simulink model "second_proto"  (R2023a)
settings: Solver=VariableStepAuto  StartTime=0.0  StopTime=10.0  RelTol=1e-3
settings Model: Creator=Алексей  LastModifiedBy=Алексей

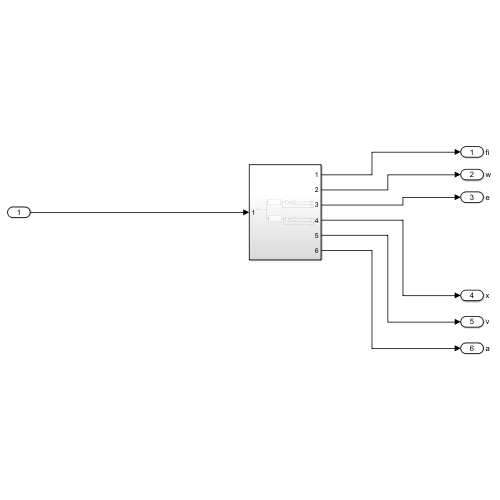
[thumbnail: Simulink's stored preview of the top-level diagram]
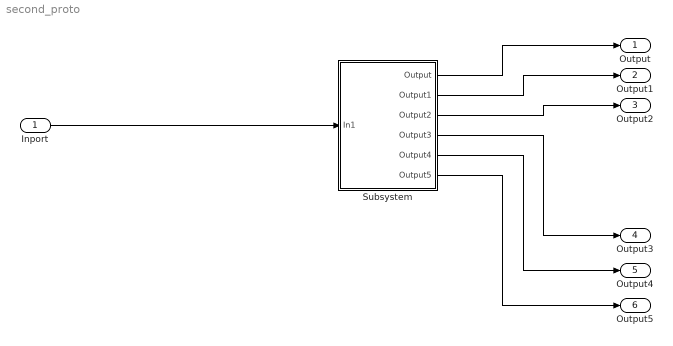
== system second_proto ==
  Inport : Inport
  Subsystem : Subsystem
  Output : Outport  SignalName=fi
  Output1 : Outport  Port=2  SignalName=w
  Output2 : Outport  Port=3  SignalName=e
  Output3 : Outport  Port=4  SignalName=x
  Output4 : Outport  Port=5  SignalName=v
  Output5 : Outport  Port=6  SignalName=a
  wires:
  Inport/1 -> Subsystem/1(In1)
  Subsystem/1(Output) -> Output/1
  Subsystem/2(Output1) -> Output1/1
  Subsystem/3(Output2) -> Output2/1
  Subsystem/4(Output3) -> Output3/1
  Subsystem/5(Output4) -> Output4/1
  Subsystem/6(Output5) -> Output5/1

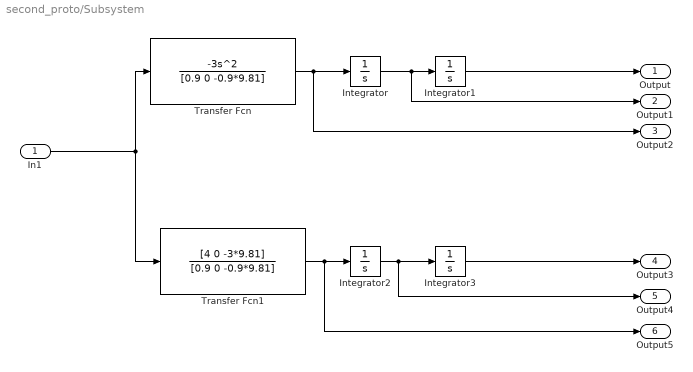
== system second_proto/Subsystem ==
  In1 : Inport
  Integrator : Integrator
  Integrator1 : Integrator  InitialCondition=5
  Integrator2 : Integrator
  Integrator3 : Integrator
  Transfer Fcn : TransferFcn  Numerator=[-3 0 0]  Denominator=[0.9 0 -0.9*9.81]
  Transfer Fcn1 : TransferFcn  Numerator=[4 0 -3*9.81]  Denominator=[0.9 0 -0.9*9.81]
  Output : Outport
  Output1 : Outport  Port=2
  Output2 : Outport  Port=3
  Output3 : Outport  Port=4
  Output4 : Outport  Port=5
  Output5 : Outport  Port=6
  wires:
  Integrator1/1 -> Output/1
  Integrator/1 -> Output1/1, Integrator1/1
  Transfer Fcn/1 -> Output2/1, Integrator/1
  Transfer Fcn1/1 -> Output5/1, Integrator2/1
  In1/1 -> Transfer Fcn1/1, Transfer Fcn/1
  Integrator3/1 -> Output3/1
  Integrator2/1 -> Output4/1, Integrator3/1
